simulink model "Temp"  (Simulink 5.1)
settings: Solver=ode4  StartTime=0.0  StopTime=8  FixedStep=1  RelTol=1e-3
libraries: simulink x2
settings Model: LastModifiedBy=清华同方  BooleanDataType=on  ProdHWDeviceType=Microprocessor

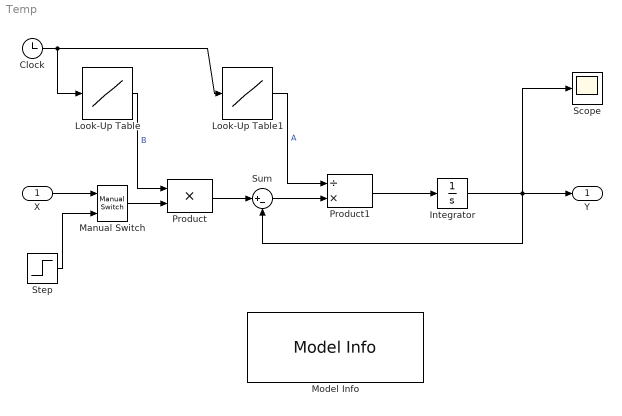
== system Temp ==
  X : Inport
  Clock : Clock
      settings: Decimation=10
  Integrator : Integrator
  Look-Up Table : Lookup  InputValues=[1:1:5]  OutputValues=[5 8 6 2 3]  SaturateOnIntegerOverflow=on
  Look-Up Table1 : Lookup  InputValues=[1:1:5]  OutputValues=[6 5 2 4 1]  SaturateOnIntegerOverflow=on
  Manual Switch : simulink/Signal Routing/Manual Switch  sw=0  action=0
  Model Info : simulink/Model-Wide Utilities/Model Info  InitialBlockCM=None  BlockCM=None  Frame=on  DisplayStringWithTags=|  HorizontalTextAlignment=Center  LeftAlignmentValue=0.5  SourceBlockDiagram=Temp  TagMaxNumber=20
      | 输入：X
      | 输出：Y
      | 参数改变根据你的需要
      | 按照插值方法给出。
  Product : Product  SaturateOnIntegerOverflow=on
  Product1 : Product  Inputs=/*  SaturateOnIntegerOverflow=on
  Scope : Scope
  Step : Step  SampleTime=0
  Sum : Sum  Inputs=|+-  SaturateOnIntegerOverflow=on
  Y : Outport
  wires:
  Look-Up Table/1 -> Product/1  "B"
  Product/1 -> Sum/1
  Sum/1 -> Product1/2
  Look-Up Table1/1 -> Product1/1  "A"
  Product1/1 -> Integrator/1
  Integrator/1 -> Sum/2, Y/1, Scope/1
  Clock/1 -> Look-Up Table/1, Look-Up Table1/1
  X/1 -> Manual Switch/1
  Step/1 -> Manual Switch/2
  Manual Switch/1 -> Product/2
